simulink model "SystemmodellingPlanB"  (R2019b)
settings: Solver=VariableStepAuto  StartTime=0.0  StopTime=10.0  RelTol=1e-3
undefined symbols (not defined in the file): c_pitch_ref, Dm, Dt, g, Jp, K, km, Kr, kt, Lm, Mb, pitch_ref, Rm, s_pitch_ref, Vdc0, Vdc1
settings Model: Creator=laptop  LastModifiedBy=laptop

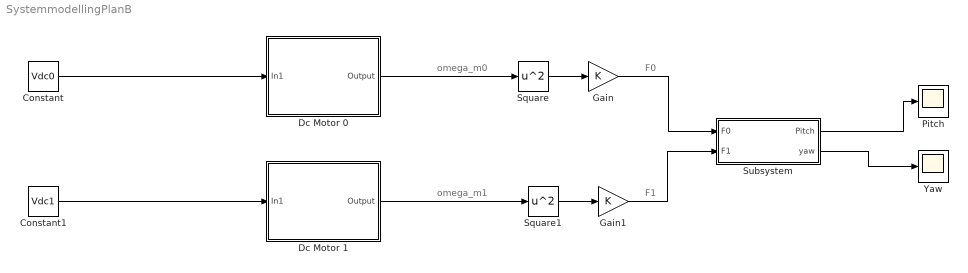
== system SystemmodellingPlanB ==
  note: F1
  note: omega_m1
  note: F0
  note: omega_m0
  Constant : Constant  Value=Vdc0
  Constant1 : Constant  Value=Vdc1
  Dc Motor 0 : Subsystem
  Dc Motor 1 : Subsystem
  Gain : Gain  Gain=K
  Gain1 : Gain  Gain=K
  Pitch : Scope
  Square : Math  Operator=square  SignedPower=off  SaturateOnIntegerOverflow=on
  Square1 : Math  Operator=square  SignedPower=off  SaturateOnIntegerOverflow=on
  Subsystem : Subsystem
  Yaw : Scope
  wires:
  Constant/1 -> Dc Motor 0/1(In1)
  Constant1/1 -> Dc Motor 1/1(In1)
  Dc Motor 0/1(Output) -> Square/1
  Square/1 -> Gain/1
  Gain/1 -> Subsystem/1(F0)
  Dc Motor 1/1(Output) -> Square1/1
  Square1/1 -> Gain1/1
  Gain1/1 -> Subsystem/2(F1)
  Subsystem/1(Pitch) -> Pitch/1
  Subsystem/2("yaw ") -> Yaw/1

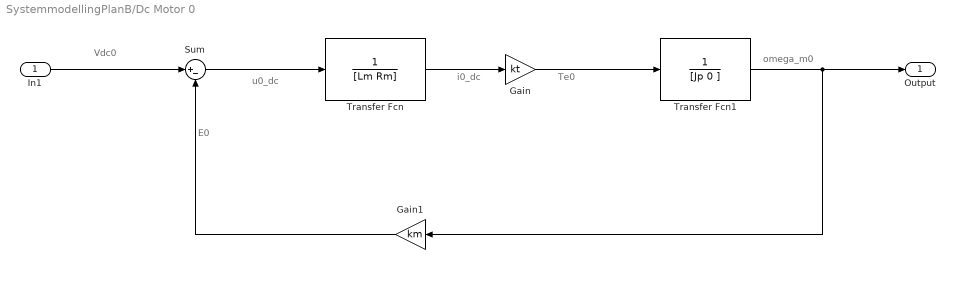
== system SystemmodellingPlanB/Dc Motor 0 ==
  note: omega_m0
  note: E0
  note: Te0
  note: i0_dc
  note: Vdc0
  note: u0_dc
  In1 : Inport
  Gain : Gain  Gain=kt
  Gain1 : Gain  Gain=km
  Sum : Sum  Inputs=|+-
  Transfer Fcn : TransferFcn  Denominator=[Lm Rm]
  Transfer Fcn1 : TransferFcn  Denominator=[Jp 0 ]
  Output : Outport
  wires:
  In1/1 -> Sum/1
  Sum/1 -> Transfer Fcn/1
  Transfer Fcn1/1 -> Output/1, Gain1/1
  Gain1/1 -> Sum/2
  Transfer Fcn/1 -> Gain/1
  Gain/1 -> Transfer Fcn1/1

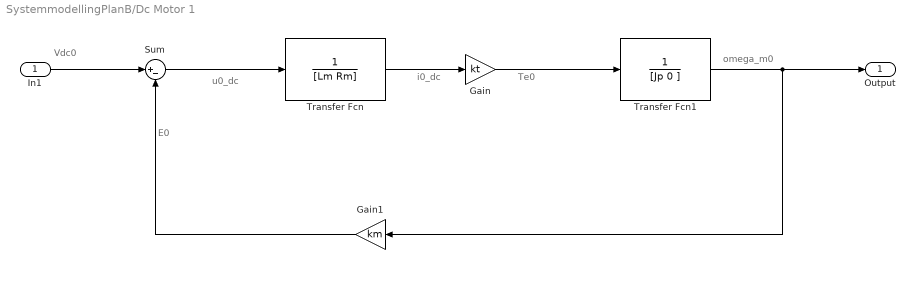
== system SystemmodellingPlanB/Dc Motor 1 ==
  note: omega_m0
  note: E0
  note: Te0
  note: i0_dc
  note: Vdc0
  note: u0_dc
  In1 : Inport
  Gain : Gain  Gain=kt
  Gain1 : Gain  Gain=km
  Sum : Sum  Inputs=|+-
  Transfer Fcn : TransferFcn  Denominator=[Lm Rm]
  Transfer Fcn1 : TransferFcn  Denominator=[Jp 0 ]
  Output : Outport
  wires:
  In1/1 -> Sum/1
  Sum/1 -> Transfer Fcn/1
  Transfer Fcn1/1 -> Output/1, Gain1/1
  Gain1/1 -> Sum/2
  Transfer Fcn/1 -> Gain/1
  Gain/1 -> Transfer Fcn1/1

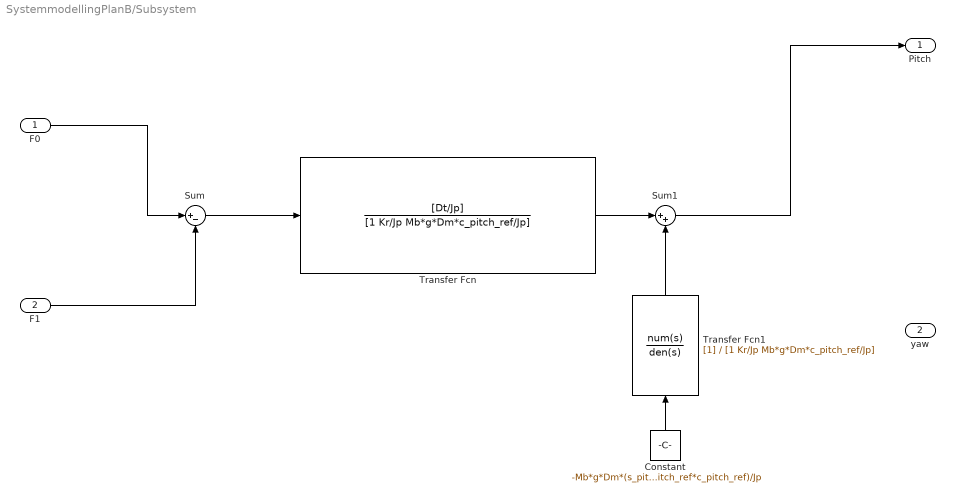
== system SystemmodellingPlanB/Subsystem ==
  F0 : Inport
  F1 : Inport  Port=2
  Constant : Constant  Value=-Mb*g*Dm*(s_pitch_ref - pitch_ref*c_pitch_ref)/Jp
  Sum : Sum  Inputs=|+-
  Sum1 : Sum  Inputs=|++
  Transfer Fcn : TransferFcn  Numerator=[Dt/Jp]  Denominator=[1 Kr/Jp Mb*g*Dm*c_pitch_ref/Jp]
  Transfer Fcn1 : TransferFcn  Denominator=[1 Kr/Jp Mb*g*Dm*c_pitch_ref/Jp]
  Pitch : Outport
  "yaw " : Outport  Port=2
  wires:
  F0/1 -> Sum/1
  F1/1 -> Sum/2
  Sum/1 -> Transfer Fcn/1
  Transfer Fcn/1 -> Sum1/1
  Transfer Fcn1/1 -> Sum1/2
  Constant/1 -> Transfer Fcn1/1
  Sum1/1 -> Pitch/1
